simulink model "gtcs_model_workbench"  (R2021a)
settings: Solver=VariableStepAuto  StartTime=0.0  StopTime=20  RelTol=1e-3
InitFcn:
  | load('param_motor.mat');
  | load('param_controller.mat');
values from neighbouring files (symbols this model uses):
  K_t = 0.0375    [param_motor.mat]
  Kp_i_active_band = 500    [param_controller.mat]
  Kp_i_satur = 1000    [param_controller.mat]
  Kp_output_deadband = 0.5    [param_controller.mat]
  Kv_d = 0    [param_controller.mat]
  Kv_ff = 1    [param_controller.mat]
  Kv_i = 0.001    [param_controller.mat]
  Kv_output_saturation_max = 1.40350877193    [param_controller.mat]
  Kv_p = 1    [param_controller.mat]
libraries: fl_lib x14, nesl_utility x6, ee_lib x2, sdl_lib x2
settings Model: Creator=ANKARA-OFIS  LastModifiedBy=ANKARA-OFIS

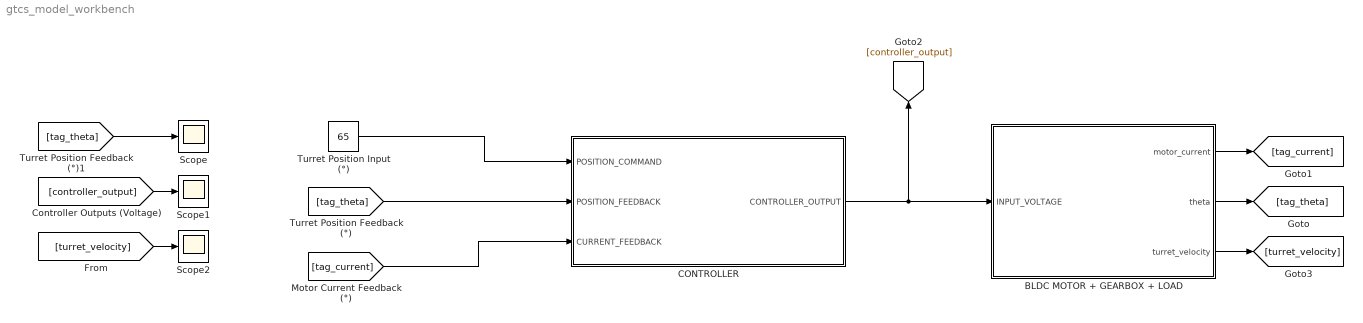
== system gtcs_model_workbench ==
  BLDC MOTOR + GEARBOX + LOAD : Subsystem
  CONTROLLER : Subsystem
  Scope : Scope
  Scope1 : Scope
  Scope2 : Scope
  Turret Position Input (°) : Constant  Value=65
  wires:
  CONTROLLER/1(CONTROLLER_OUTPUT) -> [controller_output], BLDC MOTOR + GEARBOX + LOAD/1(INPUT_VOLTAGE)
  Turret Position Input (°)/1 -> CONTROLLER/1(POSITION_COMMAND)
  BLDC MOTOR + GEARBOX + LOAD/2(theta) -> [tag_theta]
  BLDC MOTOR + GEARBOX + LOAD/1(motor_current) -> [tag_current]
  [tag_current] -> CONTROLLER/3(CURRENT_FEEDBACK)
  [tag_theta] -> CONTROLLER/2(POSITION_FEEDBACK)
  [tag_theta] -> Scope/1
  [controller_output] -> Scope1/1
  BLDC MOTOR + GEARBOX + LOAD/3(turret_velocity) -> [turret_velocity]
  [turret_velocity] -> Scope2/1

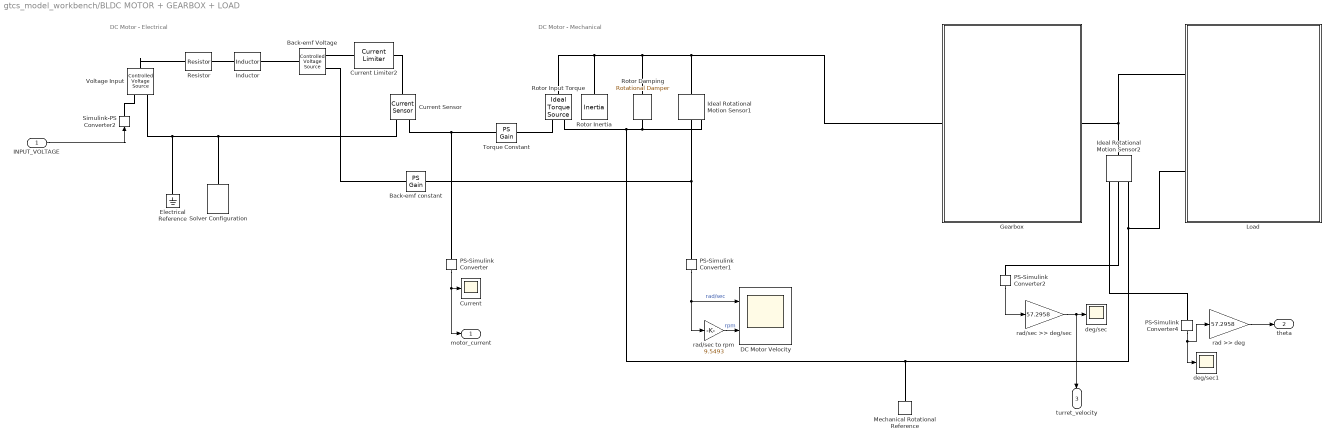
== system gtcs_model_workbench/BLDC MOTOR + GEARBOX + LOAD ==
  note: DC Motor - Mechanical
  note: DC Motor - Electrical
  INPUT_VOLTAGE : Inport
  Back-emf Voltage : fl_lib/Electrical/Electrical Sources/Controlled Voltage Source
  Back-emf constant : fl_lib/Physical Signals/Functions/PS Gain  gain=0.04 V*s/rad
  Current : Scope
  Current Limiter2 : ee_lib/Semiconductors & Converters/Current Limiter  iLim=80 A  vLim=0.1 V  gLim=1e-3 1/Ohm  thermal_mass=100 J/K  initial_temperature=298.15 K
      settings: SourceProductBaseCode=PS  InternalSimscapePortConfiguration="{\"Bottom\":[],\"Left\":[{\"id\":\"p\",\"label\":\"+\",\"type\":\"foundation.electrical.electrical\"}],\"Right\":[{\"id\":\"n\",\"label\":\"-\",\"type\":\"foundation.electrical.electrical\"}],\"Top\":[]}"
  Current Sensor : fl_lib/Electrical/Electrical Sensors/Current Sensor
  DC Motor Velocity : Scope  NumInputPorts=2
  Electrical Reference : fl_lib/Electrical/Electrical Elements/Electrical Reference
  Gearbox : Subsystem
  Ideal Rotational Motion Sensor1 : fl_lib/Mechanical/Mechanical Sensors/Ideal Rotational Motion Sensor  wrap_angle=simscape.enum.onoff.on  offset=0 rad
  Ideal Rotational Motion Sensor2 : fl_lib/Mechanical/Mechanical Sensors/Ideal Rotational Motion Sensor  wrap_angle=simscape.enum.onoff.off  offset=0 rad
  Inductor : ee_lib/Passive/Inductor  l=18e-6 H  L_tol=20  enable_L_tol=0  tol_distribution=1  nSigma=4  r=0 Ohm  g=1e-9 1/Ohm  enable_operating_limits=0  operating_limit_action=2  max_working_current=1 A  power_rating=1 W  enable_faults=0  fault_action=1  lambdaPercent=50  k_faulted=0.9999  turnsShort=0  openCct=0  groundShort=0  groundShortG=0 1/Ohm  tau_fault=1e-3 s  enable_temporal_fault=0  t_fault=1 s  enable_behavioral_fault=0  max_permissible_voltage=100 V  n_fail_on_voltage=1  max_permissible_current=1 A  t_fail_on_current=1 s  i_L_specify=off  i_L_priority=High  i_L=0 A  i_L_nominal_specify=off  i_L_nominal_unit=A  i_L_nominal_value=1
  Load : Subsystem
  Mechanical Rotational Reference : fl_lib/Mechanical/Rotational Elements/Mechanical Rotational Reference
  PS-Simulink Converter{,1..2,4} (4 alike) : nesl_utility/PS-Simulink Converter  PhysicalDomain=network_engine_domain  SubClassName=ps_output  LeftPortType=input  RightPortType=output  PseudoPeriodic=off  Frequencies=[]  Unit=inherit  AffineConversion=off
      settings: SourceProductBaseCode=PW,SS
  Resistor : fl_lib/Electrical/Electrical Elements/Resistor  R=45e-03 Ohm  i_specify=off  i_priority=None  i=0 A  i_nominal_specify=off  i_nominal_unit=A  i_nominal_value=1  v_specify=off  v_priority=None  v=0 V  v_nominal_specify=off  v_nominal_unit=V  v_nominal_value=1
  Rotor Damping : fl_lib/Mechanical/Rotational Elements/Rotational Damper  D=0.0001 N*m/(rad/s)  w_specify=off  w_priority=None  w=0 rad/s  w_nominal_specify=off  w_nominal_unit=rad/s  w_nominal_value=1  t_specify=off  t_priority=None  t=0 N*m  t_nominal_specify=off  t_nominal_unit=N*m  t_nominal_value=1
  Rotor Inertia : fl_lib/Mechanical/Rotational Elements/Inertia  inertia=100 kg*mm^2  num_ports=foundation.enum.numPorts2.one  w_specify=off  w_priority=High  w=0 rad/s  w_nominal_specify=off  w_nominal_unit=rad/s  w_nominal_value=1  t_specify=off  t_priority=None  t=0 N*m  t_nominal_specify=off  t_nominal_unit=N*m  t_nominal_value=1
  Rotor Input Torque : fl_lib/Mechanical/Mechanical Sources/Ideal Torque Source
  Simulink-PS Converter2 : nesl_utility/Simulink-PS Converter  PhysicalDomain=network_engine_domain  SubClassName=ps_input  LeftPortType=input  RightPortType=output  PseudoPeriodic=off  Frequencies=[]  NoiseDistribution=none  NoiseParameters=[]  Unit=1  AffineConversion=off  FilteringAndDerivatives=provide  SimscapeFilterOrder=1  InputFilterTimeConstant=0.001  UdotUserProvided=0
      settings: SourceProductBaseCode=PW,SS
  Solver Configuration : nesl_utility/Solver Configuration  PhysicalDomain=network_engine_domain  SubClassName=solver  LeftPortType=input  RightPortType=generic  Tones=[]  Harmonics=[]  SimulateNoise=off  Profile=off  UseLocalSampling=off  EnableSwitchedLinearOptims=on  FrequencyDomain=off  UseCCode=off  RelTol=0.001  AbsTol=1e-06  MinStep=1e-09  ToWorkspace=off  RevertToSquareIcSolve=off  NumHomotopyIterations=100  PhasorMode=off  PhasorModeNumHarmonics=1  DoDC=off  ResidualTolerance=1e-09  UseLocalSolver=off  LocalSolverChoice=NE_BACKWARD_EULER_ADVANCER  LocalSolverSampleTime=0.001  DoFixedCost=off  MaxNonlinIter=3  MaxModeIter=2  ComputeImpulses=off  ImpulseIterations=2  LinearAlgebra=auto  EquationFormulation=NE_TIME_EF  DelaysMemoryBudget=1024  AutomaticFiltering=on  FilteringTimeConstant=0.001  PartitionStorageMethod=AS_NEEDED  PartitionMemoryBudget=1024  PartitionMethod=ROBUST
      settings: SourceProductBaseCode=PW,SS
  Torque Constant : fl_lib/Physical Signals/Functions/PS Gain  gain=K_t N*m/A
  Voltage Input : fl_lib/Electrical/Electrical Sources/Controlled Voltage Source
  deg/sec : Scope
  deg/sec1 : Scope
  rad >> deg : Gain  Gain=57.2958
  rad/sec >> deg/sec : Gain  Gain=57.2958
  rad/sec to rpm : Gain  Gain=9.5493
  motor_current : Outport
  theta : Outport  Port=2
  turret_velocity : Outport  Port=3
  wires:
  PS-Simulink Converter2/1 -> rad/sec >> deg/sec/1
  INPUT_VOLTAGE/1 -> Simulink-PS Converter2/1
  PS-Simulink Converter/1 -> motor_current/1, Current/1
  PS-Simulink Converter1/1 -> DC Motor Velocity/1, rad/sec to rpm/1  "rad/sec"
  rad/sec to rpm/1 -> DC Motor Velocity/2  "rpm"
  rad/sec >> deg/sec/1 -> turret_velocity/1, deg/sec/1
  PS-Simulink Converter4/1 -> rad >> deg/1, deg/sec1/1
  rad >> deg/1 -> theta/1
  connections:
  Rotor Damping/LConn1 -- Rotor Input Torque/LConn1 -- Rotor Inertia/LConn1 -- Gearbox/LConn1 -- Ideal Rotational Motion Sensor1/LConn1
  Mechanical Rotational Reference/LConn1 -- Rotor Damping/RConn1 -- Ideal Rotational Motion Sensor1/RConn1 -- Rotor Input Torque/RConn2 -- Ideal Rotational Motion Sensor2/RConn1 -- Load/LConn2
  Ideal Rotational Motion Sensor2/RConn2 -- PS-Simulink Converter2/LConn1
  Torque Constant/RConn1 -- Rotor Input Torque/RConn1
  Ideal Rotational Motion Sensor1/RConn2 -- PS-Simulink Converter1/LConn1 -- Back-emf constant/LConn1
  Voltage Input/RConn1 -- Simulink-PS Converter2/RConn1
  Resistor/RConn1 -- Inductor/LConn1
  Current Limiter2/RConn1 -- Current Sensor/LConn1
  Voltage Input/LConn1 -- Resistor/LConn1
  Back-emf Voltage/RConn2 -- Current Limiter2/LConn1
  Torque Constant/LConn1 -- Current Sensor/RConn1 -- PS-Simulink Converter/LConn1
  Back-emf constant/RConn1 -- Back-emf Voltage/RConn1
  Back-emf Voltage/LConn1 -- Inductor/RConn1
  Electrical Reference/LConn1 -- Voltage Input/RConn2 -- Solver Configuration/RConn1 -- Current Sensor/RConn2
  Gearbox/RConn1 -- Load/LConn1 -- Ideal Rotational Motion Sensor2/LConn1
  Ideal Rotational Motion Sensor2/RConn3 -- PS-Simulink Converter4/LConn1

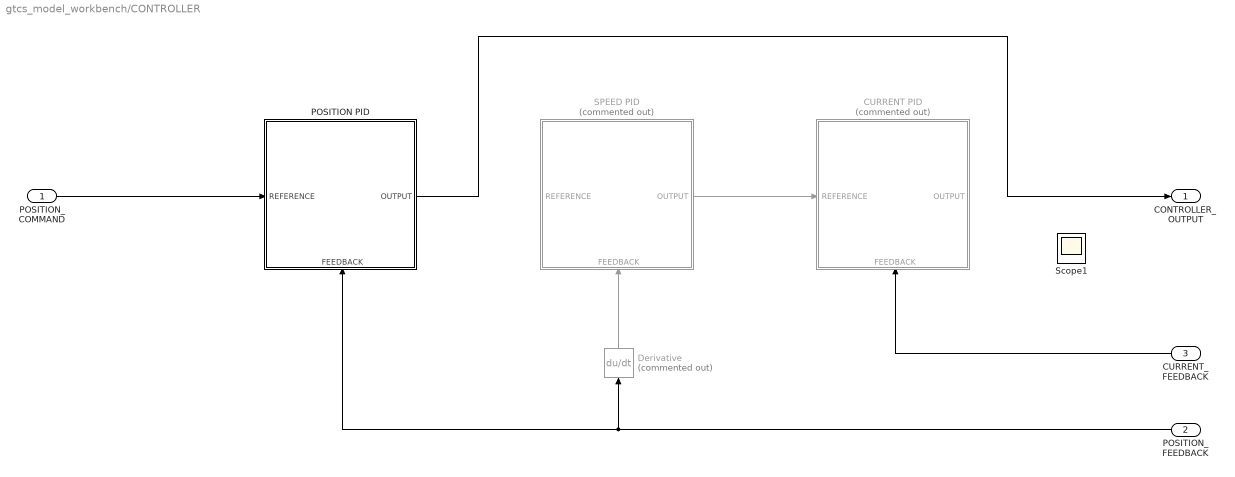
== system gtcs_model_workbench/CONTROLLER ==
  POSITION_COMMAND : Inport
  POSITION_FEEDBACK : Inport  Port=2
  CURRENT_FEEDBACK : Inport  Port=3
  CURRENT PID : Subsystem  Commented=on
      settings: PortSchema="{\"entries\":[{\"content\":{\"sides\":[{\"content\":{\"connectorIds\":[\"In1\"]},\"type\":\"ConnectorPlacement.EquallySpacedRectSide\",\"uuid\":\"40c65be9-b241-43d3-b74e-061528d6863f\"},{\"content\":{\"connectorIds\":[\"Out1\"],\"side\":\"RIGHT\"},\"type\":\"ConnectorPlacement.EquallySpacedRectSide\",\"uuid\":\"f0c37777-6186-40ca-93fa-111567e4da2a\"},{\"content\":{\"connectorIds\":[],\"side\":\"TOP\"},\"type\":\"ConnectorPlacement.EquallySpacedRectSide\",\"uuid\":\"f72b91dc-29bd-47db-bfb1-a15381258f12\"},{\"content\":{\"connectorIds\":[\"In2\"],\"side\":\"BOTTOM\"},\"type\":\"ConnectorPlacement.EquallySpacedRectSide\",\"uuid\":\"2008c998-139c-4ab5-8b80-fe5598144eb1\"}]},\"type\":\"ConnectorPlacement.EquallySpacedConnector\",\"uuid\":\"6c18c1ed-cfc3-452d-a661-af16ec8cef93\"}],\"packageUris\":[\"http://schema.mathworks.com/mf0/Connector/R2020b\"],\"version\":\"1.0\"}"
  Derivative : Derivative  Commented=on
  POSITION PID : Subsystem
      settings: PortSchema="{\"entries\":[{\"content\":{\"sides\":[{\"content\":{\"connectorIds\":[\"In1\"]},\"type\":\"ConnectorPlacement.EquallySpacedRectSide\",\"uuid\":\"40c65be9-b241-43d3-b74e-061528d6863f\"},{\"content\":{\"connectorIds\":[\"Out1\"],\"side\":\"RIGHT\"},\"type\":\"ConnectorPlacement.EquallySpacedRectSide\",\"uuid\":\"f0c37777-6186-40ca-93fa-111567e4da2a\"},{\"content\":{\"connectorIds\":[],\"side\":\"TOP\"},\"type\":\"ConnectorPlacement.EquallySpacedRectSide\",\"uuid\":\"f72b91dc-29bd-47db-bfb1-a15381258f12\"},{\"content\":{\"connectorIds\":[\"In2\"],\"side\":\"BOTTOM\"},\"type\":\"ConnectorPlacement.EquallySpacedRectSide\",\"uuid\":\"2008c998-139c-4ab5-8b80-fe5598144eb1\"}]},\"type\":\"ConnectorPlacement.EquallySpacedConnector\",\"uuid\":\"6c18c1ed-cfc3-452d-a661-af16ec8cef93\"}],\"packageUris\":[\"http://schema.mathworks.com/mf0/Connector/R2020b\"],\"version\":\"1.0\"}"
  SPEED PID : Subsystem  Commented=on
      settings: PortSchema="{\"entries\":[{\"content\":{\"sides\":[{\"content\":{\"connectorIds\":[\"In1\"]},\"type\":\"ConnectorPlacement.EquallySpacedRectSide\",\"uuid\":\"40c65be9-b241-43d3-b74e-061528d6863f\"},{\"content\":{\"connectorIds\":[\"Out1\"],\"side\":\"RIGHT\"},\"type\":\"ConnectorPlacement.EquallySpacedRectSide\",\"uuid\":\"f0c37777-6186-40ca-93fa-111567e4da2a\"},{\"content\":{\"connectorIds\":[],\"side\":\"TOP\"},\"type\":\"ConnectorPlacement.EquallySpacedRectSide\",\"uuid\":\"f72b91dc-29bd-47db-bfb1-a15381258f12\"},{\"content\":{\"connectorIds\":[\"In2\"],\"side\":\"BOTTOM\"},\"type\":\"ConnectorPlacement.EquallySpacedRectSide\",\"uuid\":\"2008c998-139c-4ab5-8b80-fe5598144eb1\"}]},\"type\":\"ConnectorPlacement.EquallySpacedConnector\",\"uuid\":\"6c18c1ed-cfc3-452d-a661-af16ec8cef93\"}],\"packageUris\":[\"http://schema.mathworks.com/mf0/Connector/R2020b\"],\"version\":\"1.0\"}"
  Scope1 : Scope
  CONTROLLER_OUTPUT : Outport
  wires:
  Derivative/1 -> SPEED PID/2(FEEDBACK)
  CURRENT_FEEDBACK/1 -> CURRENT PID/2(FEEDBACK)
  SPEED PID/1(OUTPUT) -> CURRENT PID/1(REFERENCE)
  POSITION_FEEDBACK/1 -> POSITION PID/2(FEEDBACK), Derivative/1
  POSITION_COMMAND/1 -> POSITION PID/1(REFERENCE)
  POSITION PID/1(OUTPUT) -> CONTROLLER_OUTPUT/1

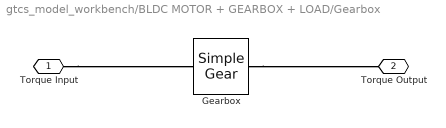
== system gtcs_model_workbench/BLDC MOTOR + GEARBOX + LOAD/Gearbox ==
  Gearbox : sdl_lib/Gears/Simple Gear  ratio=435.6  rotation_direction=sdl.enum.shaftOutputDirection.same  friction_model=sdl.enum.gear_efficiencies_load.off  mu_visc=[0, 0] N*m/(rad/s)  T_noload=0.1 N*m  T_nom=5 N*m  efficiency_nom=0.8  efficiency=0.8  temperature_TLU=[280, 300, 320] K  load_TLU=[1, 5, 10] N*m  efficiency_TLU=[.95, .9, .85]  efficiency_TLU2=[.85, .8, .75; .95, .9, .85; .85, .8, .7]  w_thr=0.01 rad/s  pwr_thr=0.001 W  thermal_mass=50 J/K  enable_faults=simscape.enum.onoff.off  efficiency_fault=0.05  external_fault=simscape.enum.onoff.off  temporal_fault=simscape.enum.onoff.off  fault_time=5 s  fault_angles=pi / 12 rad  report_fault=simscape.enum.assert.action.none  temperature_specify=off  temperature_priority=High  temperature=300 K  temperature_nominal_specify=off  temperature_nominal_unit=K  temperature_nominal_value=1
  Torque Input : PMIOPort  Side=Left
  Torque Output : PMIOPort  Port=2  Side=Right
  connections:
  Gearbox/RConn1 -- Torque Output/RConn1
  Torque Input/RConn1 -- Gearbox/LConn1

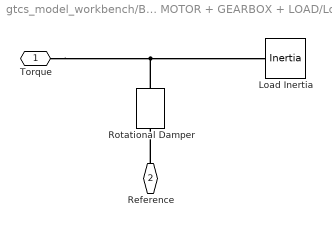
== system gtcs_model_workbench/BLDC MOTOR + GEARBOX + LOAD/Load ==
  Load Inertia : fl_lib/Mechanical/Rotational Elements/Inertia  inertia=257 kg*m^2  num_ports=foundation.enum.numPorts2.one  w_specify=off  w_priority=High  w=0 rad/s  w_nominal_specify=off  w_nominal_unit=rad/s  w_nominal_value=1  t_specify=off  t_priority=None  t=0 N*m  t_nominal_specify=off  t_nominal_unit=N*m  t_nominal_value=1
  Rotational Damper : sdl_lib/Couplings & Drives/Springs & Dampers/Rotational Damper  D=0.1 N*m/(rad/s)  enable_faults=0  b_fault=100 N*m/(rad/s)  temporal_fault=0  fault_time=5 s  shock_fault=0  acceleration_limit=100 rad/s^2  shock_limit=1  report_fault=1
      settings: SourceProductBaseCode=LD
  Torque : PMIOPort  Side=Left
  Reference : PMIOPort  Port=2  Side=Left
  connections:
  Torque/RConn1 -- Rotational Damper/LConn1 -- Load Inertia/LConn1
  Reference/RConn1 -- Rotational Damper/RConn1

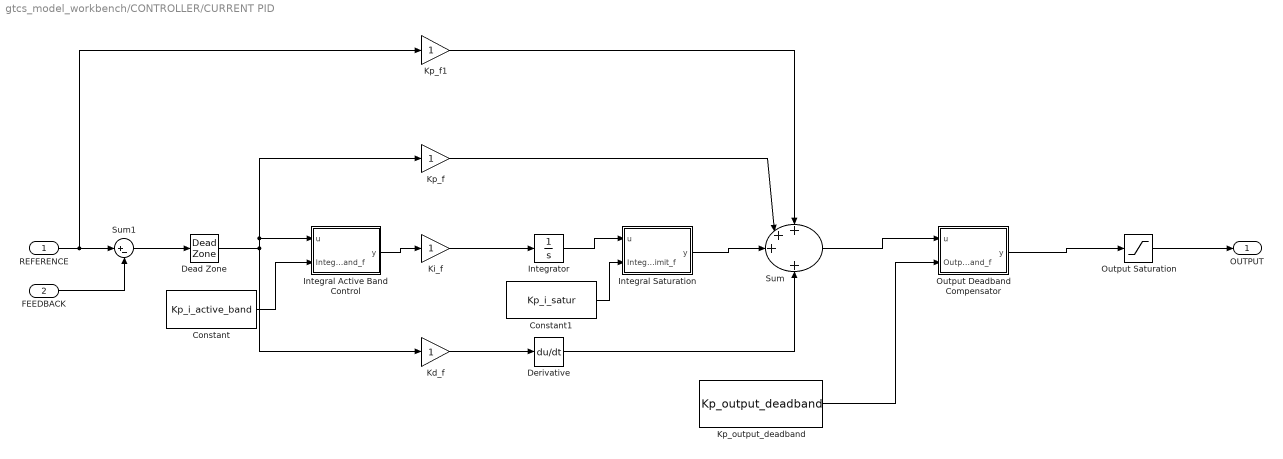
== system gtcs_model_workbench/CONTROLLER/CURRENT PID ==
  REFERENCE : Inport
  FEEDBACK : Inport  Port=2
  Constant : Constant  Value=Kp_i_active_band
  Constant1 : Constant  Value=Kp_i_satur
  Dead Zone : DeadZone  SaturateOnIntegerOverflow=on
  Derivative : Derivative
  Integral Active Band Control : MATLAB Function  TreatAsAtomicUnit=on
  Integral Saturation : MATLAB Function  TreatAsAtomicUnit=on
  Integrator : Integrator
  Kd_f : Gain
  Ki_f : Gain
  Kp_f : Gain
  Kp_f1 : Gain
  Kp_output_deadband : Constant  Value=Kp_output_deadband
  Output Deadband Compensator : MATLAB Function  TreatAsAtomicUnit=on
  Output Saturation : Saturate
  Sum : Sum  Inputs=+++|+
  Sum1 : Sum  Inputs=|+-
  OUTPUT : Outport
  wires:
  Integrator/1 -> Integral Saturation/1(u)
  Integral Saturation/1(y) -> Sum/3
  Output Deadband Compensator/1(y) -> Output Saturation/1
  Ki_f/1 -> Integrator/1
  Kd_f/1 -> Derivative/1
  Derivative/1 -> Sum/4
  Kp_f1/1 -> Sum/1
  Output Saturation/1 -> OUTPUT/1
  Integral Active Band Control/1(y) -> Ki_f/1
  Kp_f/1 -> Sum/2
  Sum/1 -> Output Deadband Compensator/1(u)
  FEEDBACK/1 -> Sum1/2
  REFERENCE/1 -> Kp_f1/1, Sum1/1
  Sum1/1 -> Dead Zone/1
  Dead Zone/1 -> Kp_f/1, Integral Active Band Control/1(u), Kd_f/1
  Constant/1 -> Integral Active Band Control/2(IntegralActiveBand_f)
  Constant1/1 -> Integral Saturation/2(IntegralLimit_f)
  Kp_output_deadband/1 -> Output Deadband Compensator/2(OutputDeadband_f)

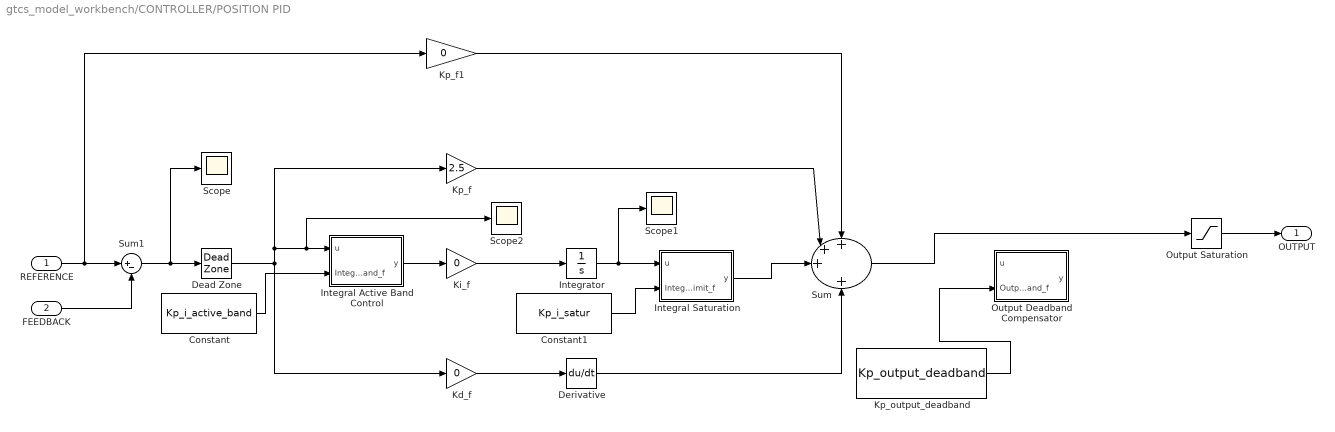
== system gtcs_model_workbench/CONTROLLER/POSITION PID ==
  REFERENCE : Inport
  FEEDBACK : Inport  Port=2
  Constant : Constant  Value=Kp_i_active_band
  Constant1 : Constant  Value=Kp_i_satur
  Dead Zone : DeadZone  SaturateOnIntegerOverflow=on
  Derivative : Derivative
  Integral Active Band Control : MATLAB Function  TreatAsAtomicUnit=on
  Integral Saturation : MATLAB Function  TreatAsAtomicUnit=on
  Integrator : Integrator
  Kd_f : Gain  Gain=0
  Ki_f : Gain  Gain=0
  Kp_f : Gain  Gain=2.5
  Kp_f1 : Gain  Gain=0
  Kp_output_deadband : Constant  Value=Kp_output_deadband
  Output Deadband Compensator : MATLAB Function  TreatAsAtomicUnit=on
  Output Saturation : Saturate  UpperLimit=28  LowerLimit=-28
  Scope : Scope
  Scope1 : Scope
  Scope2 : Scope
  Sum : Sum  Inputs=+++|+
  Sum1 : Sum  Inputs=|+-
  OUTPUT : Outport
  wires:
  Integrator/1 -> Scope1/1, Integral Saturation/1(u)
  Integral Saturation/1(y) -> Sum/3
  Ki_f/1 -> Integrator/1
  Kd_f/1 -> Derivative/1
  Derivative/1 -> Sum/4
  Kp_f1/1 -> Sum/1
  Output Saturation/1 -> OUTPUT/1
  Integral Active Band Control/1(y) -> Ki_f/1
  Kp_f/1 -> Sum/2
  FEEDBACK/1 -> Sum1/2
  REFERENCE/1 -> Kp_f1/1, Sum1/1
  Sum1/1 -> Scope/1, Dead Zone/1
  Dead Zone/1 -> Kp_f/1, Scope2/1, Integral Active Band Control/1(u), Kd_f/1
  Constant/1 -> Integral Active Band Control/2(IntegralActiveBand_f)
  Constant1/1 -> Integral Saturation/2(IntegralLimit_f)
  Kp_output_deadband/1 -> Output Deadband Compensator/2(OutputDeadband_f)
  Sum/1 -> Output Saturation/1

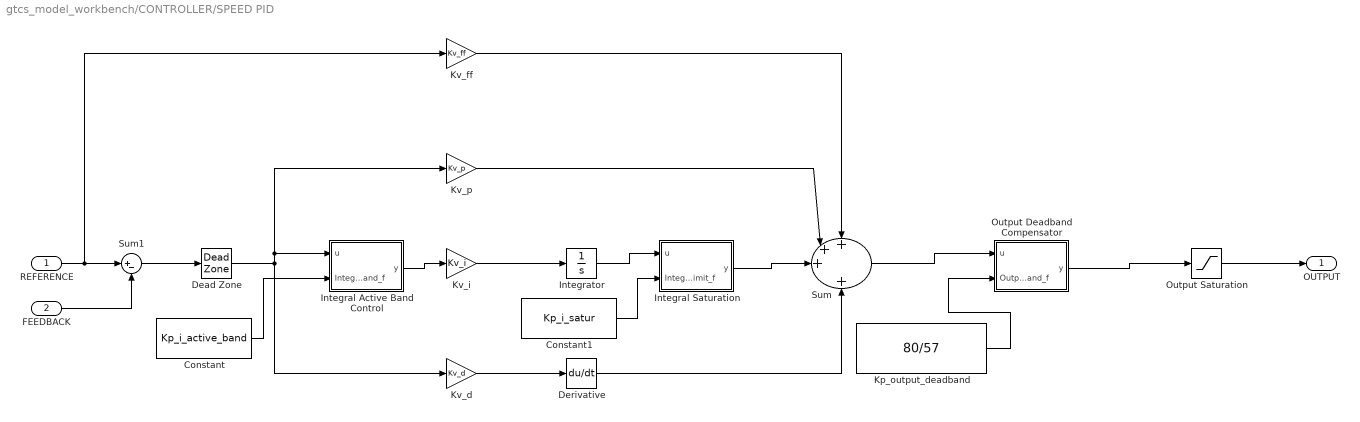
== system gtcs_model_workbench/CONTROLLER/SPEED PID ==
  REFERENCE : Inport
  FEEDBACK : Inport  Port=2
  Constant : Constant  Value=Kp_i_active_band
  Constant1 : Constant  Value=Kp_i_satur
  Dead Zone : DeadZone  SaturateOnIntegerOverflow=on
  Derivative : Derivative
  Integral Active Band Control : MATLAB Function  TreatAsAtomicUnit=on
  Integral Saturation : MATLAB Function  TreatAsAtomicUnit=on
  Integrator : Integrator
  Kp_output_deadband : Constant  Value=80/57
  Kv_d : Gain  Gain=Kv_d
  Kv_ff : Gain  Gain=Kv_ff
  Kv_i : Gain  Gain=Kv_i
  Kv_p : Gain  Gain=Kv_p
  Output Deadband Compensator : MATLAB Function  TreatAsAtomicUnit=on
  Output Saturation : Saturate  UpperLimit=Kv_output_saturation_max  LowerLimit=0.01
  Sum : Sum  Inputs=+++|+
  Sum1 : Sum  Inputs=|+-
  OUTPUT : Outport
  wires:
  Dead Zone/1 -> Integral Active Band Control/1(u), Kv_p/1, Kv_d/1
  Sum1/1 -> Dead Zone/1
  REFERENCE/1 -> Sum1/1, Kv_ff/1
  FEEDBACK/1 -> Sum1/2
  Sum/1 -> Output Deadband Compensator/1(u)
  Kv_p/1 -> Sum/2
  Integral Active Band Control/1(y) -> Kv_i/1
  Output Saturation/1 -> OUTPUT/1
  Kv_ff/1 -> Sum/1
  Derivative/1 -> Sum/4
  Kv_d/1 -> Derivative/1
  Kv_i/1 -> Integrator/1
  Output Deadband Compensator/1(y) -> Output Saturation/1
  Integral Saturation/1(y) -> Sum/3
  Integrator/1 -> Integral Saturation/1(u)
  Constant1/1 -> Integral Saturation/2(IntegralLimit_f)
  Kp_output_deadband/1 -> Output Deadband Compensator/2(OutputDeadband_f)
  Constant/1 -> Integral Active Band Control/2(IntegralActiveBand_f)

== matlab function gtcs_model_workbench/CONTROLLER/POSITION PID/Integral Saturation ==
  data: u input; y output; IntegralLimit_f input
function y = IntegralSaturation(u, IntegralLimit_f)
    if u==0
        multiplier = 1;
    else
        multiplier = floor(u/abs(u));
    end
    if abs(u) < IntegralLimit_f
        y = u;
    else
        y = IntegralLimit_f * multiplier;
    end
end

== matlab function gtcs_model_workbench/CONTROLLER/POSITION PID/Output Deadband Compensator ==
  data: u input; y output; OutputDeadband_f input
function y = Output_Deadband_Compensator(u, OutputDeadband_f)
    if u==0
        multiplier = 1;
    else
        multiplier = floor(u/abs(u));
    end
    if abs(u) == 0
        y = 0;
    else
        y = u + OutputDeadband_f * multiplier;
    end
end

== matlab function gtcs_model_workbench/CONTROLLER/SPEED PID/Integral Active Band Control ==
  data: u input; y output; IntegralActiveBand_f input
function y = IntegralActiveBandControl(u, IntegralActiveBand_f)
    if abs(u) <= IntegralActiveBand_f
        y = u;
    else
        y = 0;
    end
end

== matlab function gtcs_model_workbench/CONTROLLER/SPEED PID/Integral Saturation ==
  data: u input; y output; IntegralLimit_f input
function y = IntegralSaturation(u, IntegralLimit_f)
    if u==0
        multiplier = 1;
    else
        multiplier = floor(u/abs(u));
    end
    if abs(u) < IntegralLimit_f
        y = u;
    else
        y = IntegralLimit_f * multiplier;
    end
end

== matlab function gtcs_model_workbench/CONTROLLER/SPEED PID/Output Deadband Compensator ==
  data: u input; y output; OutputDeadband_f input
function y = Output_Deadband_Compensator(u, OutputDeadband_f)
    if u==0
        multiplier = 1;
    else
        multiplier = floor(u/abs(u));
    end
    if abs(u) == 0
        y = 0;
    else
        y = u + OutputDeadband_f * multiplier;
    end
end

== matlab function gtcs_model_workbench/CONTROLLER/CURRENT PID/Integral Active Band Control ==
  data: u input; y output; IntegralActiveBand_f input
function y = IntegralActiveBandControl(u, IntegralActiveBand_f)
    if abs(u) <= IntegralActiveBand_f
        y = u;
    else
        y = 0;
    end
end

== matlab function gtcs_model_workbench/CONTROLLER/CURRENT PID/Integral Saturation ==
  data: u input; y output; IntegralLimit_f input
function y = IntegralSaturation(u,IntegralLimit_f)
    if u==0
        multiplier = 1;
    else
        multiplier = floor(u/abs(u));
    end
    if abs(u) < IntegralLimit_f
        y = u;
    else
        y = IntegralLimit_f * multiplier;
    end
end

== matlab function gtcs_model_workbench/CONTROLLER/CURRENT PID/Output Deadband Compensator ==
  data: u input; y output; OutputDeadband_f input
function y = Output_Deadband_Compensator(u, OutputDeadband_f)
    if u==0
        multiplier = 1;
    else
        multiplier = floor(u/abs(u));
    end
    if abs(u) == 0
        y = 0;
    else
        y = u + OutputDeadband_f * multiplier;
    end
end

== matlab function gtcs_model_workbench/CONTROLLER/POSITION PID/Integral Active Band Control ==
  data: u input; y output; IntegralActiveBand_f input
function y = IntegralActiveBandControl(u, IntegralActiveBand_f)
    if abs(u) <= IntegralActiveBand_f
        y = u;
    else
        y = 0;
    end
end
